simulink model "proc_control_lite"  (R2024b)
settings: Solver=FixedStepAuto  StartTime=0.0  StopTime=inf  RelTol=1e-3
InitFcn:
  | InitProcControl;
StartFcn:
  | LoadParams;
model workspace (MAT data in the model file):
  SL_ROS_VariableLengthArrays_MaxSizes : object (value not decoded)
values from neighbouring files (symbols this model uses):
  A = T200Spec16V{:,3}    [InitProcControl.m]
  N = T200Spec16V{:,6}    [InitProcControl.m]
  PWM = T200Spec16V{:,1}    [InitProcControl.m]
undefined symbols (not defined in the file or in its folder): config, current_gains, DiscIntNeverNeededParam, is_mpc_alive, is_trajectory_done, motor1, motor2, motor3, motor4, motor5, motor6, motor7, motor8, MPC, mpc_mode, mpc_status, orientation, physics, pose, position, simulation, simulink, target_reached, thrusters_status, thrusters_status_SL_Info, twist
libraries: ros2lib x64, dspstat3 x24, aerolibutil x15, dspfdesign x7, simulink x5, mpclib x3, matrix_library x3, robotcorelib x2, sharedtransform x1, sharedTrackingLibrary x1
(part 3 of 3)

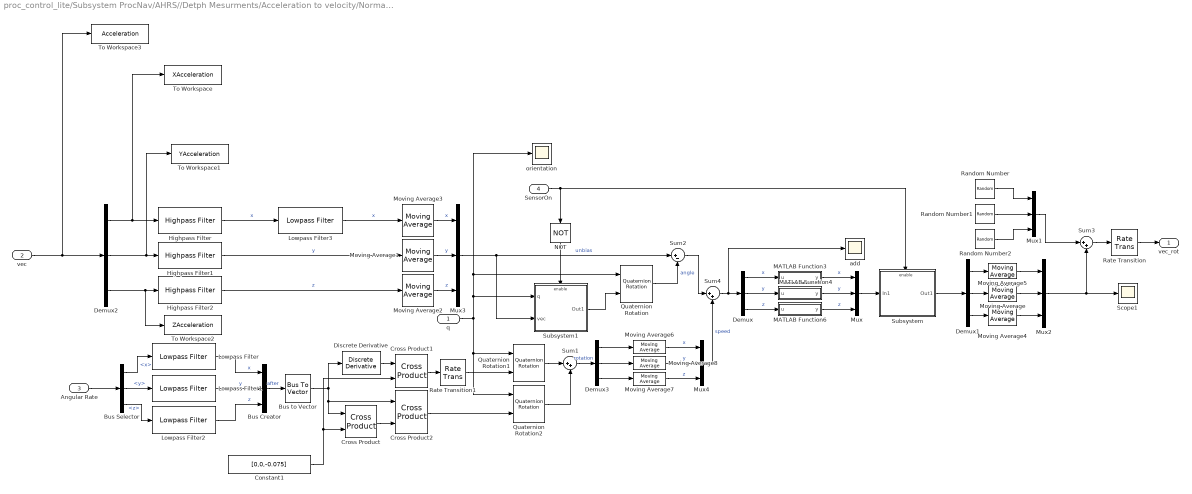
== system proc_control_lite/Subsystem ProcNav/AHRS//Detph Mesurments/Acceleration to velocity/Normal mode ==
  q : Inport
  vec : Inport  Port=2
  Angular Rate : Inport  Port=3
  SensorOn : Inport  Port=4
  Bus Creator : BusCreator  Inputs=3
  Bus Selector : BusSelector  OutputSignals=x,y,z
  Bus to Vector : BusToVector
  Constant1 : Constant  Value=[0,0,-0.075]
  Cross Product : matrix_library/Cross Product
  Cross Product1 : matrix_library/Cross Product
  Cross Product2 : matrix_library/Cross Product
  Demux{,1..3} (4 alike) : Demux  Outputs=3
  Discrete Derivative : simulink/Discrete/Discrete Derivative  gainval=1.0  ICPrevScaledInput=0.0  OutMin=[]  OutMax=[]  OutDataType=fixdt(1, 16)  OutScaling=2^-10  DoSatur=off
  Highpass Filter : dspfdesign/Highpass Filter  FilterType=IIR  DesignForMinimumOrder=on  FilterOrder=50  StopbandFrequency=0.5  PassbandFrequency=0.75  StopbandAttenuation=100  PassbandRipple=0.1  SampleRateMode=Specify on dialog  SampleRate=50  SimulateUsing=Interpreted execution  roundingMode=Floor  coeffsDataTypeStr=fixdt(1,16)
  Highpass Filter1 : dspfdesign/Highpass Filter  FilterType=IIR  DesignForMinimumOrder=on  FilterOrder=50  StopbandFrequency=0.2  PassbandFrequency=0.25  StopbandAttenuation=100  PassbandRipple=0.1  SampleRateMode=Use normalized frequency (0 to 1)  SampleRate=44100  SimulateUsing=Interpreted execution  roundingMode=Floor  coeffsDataTypeStr=fixdt(1,16)
  Highpass Filter2 : dspfdesign/Highpass Filter  FilterType=IIR  DesignForMinimumOrder=on  FilterOrder=50  StopbandFrequency=0.2  PassbandFrequency=0.25  StopbandAttenuation=100  PassbandRipple=0.1  SampleRateMode=Use normalized frequency (0 to 1)  SampleRate=44100  SimulateUsing=Interpreted execution  roundingMode=Floor  coeffsDataTypeStr=fixdt(1,16)
  Lowpass Filter{,1..3} (4 alike) : dspfdesign/Lowpass Filter  FilterType=FIR  DesignForMinimumOrder=on  FilterOrder=50  PassbandFrequency=0.10  StopbandFrequency=0.15  PassbandRipple=0.1  StopbandAttenuation=80  SampleRateMode=Use normalized frequency (0 to 1)  SampleRate=44100  SimulateUsing=Interpreted execution  roundingMode=Floor  coeffsDataTypeStr=fixdt(1,16)
  MATLAB Function3 : MATLAB Function  TreatAsAtomicUnit=on
  MATLAB Function4 : MATLAB Function  TreatAsAtomicUnit=on
  MATLAB Function6 : MATLAB Function  TreatAsAtomicUnit=on
  Moving Average : dspstat3/Moving Average  Method=Sliding window  ForgettingFactorPort=off  SpecifyWindowLength=on  WindowLength=10  OverlapLength=9  AllowArbitraryInputLength=off  ForgettingFactor=0.9  SimulateUsing=Interpreted execution
  Moving Average{1..3,6..8} (6 alike) : dspstat3/Moving Average  Method=Sliding window  ForgettingFactorPort=off  SpecifyWindowLength=on  WindowLength=5  OverlapLength=4  AllowArbitraryInputLength=off  ForgettingFactor=0.9  SimulateUsing=Interpreted execution
  Moving Average4 : dspstat3/Moving Average  Method=Sliding window  ForgettingFactorPort=off  SpecifyWindowLength=on  WindowLength=10  OverlapLength=9  AllowArbitraryInputLength=off  ForgettingFactor=0.9  SimulateUsing=Interpreted execution
  Moving Average5 : dspstat3/Moving Average  Method=Sliding window  ForgettingFactorPort=off  SpecifyWindowLength=on  WindowLength=10  OverlapLength=9  AllowArbitraryInputLength=off  ForgettingFactor=0.9  SimulateUsing=Interpreted execution
  Mux{,1..4} (5 alike) : Mux  Inputs=3
  NOT : Logic  Operator=NOT  IconShape=distinctive  AllPortsSameDT=off  OutDataTypeStr=boolean
  Quaternion Rotation : aerolibutil/Quaternion Rotation
  Quaternion Rotation1 : aerolibutil/Quaternion Rotation
  Quaternion Rotation2 : aerolibutil/Quaternion Rotation
  Random Number : RandomNumber  Variance=0.0000000001  Seed=1  SampleTime=0.02
  Random Number1 : RandomNumber  Variance=0.0000000001  Seed=525886  SampleTime=0.02
  Random Number2 : RandomNumber  Variance=0.0000000001  Seed=4  SampleTime=0.02
  Rate Transition : RateTransition  OutPortSampleTime=0.02
  Rate Transition1 : RateTransition  OutPortSampleTime=0.02
  Scope1 : Scope
  Subsystem : Subsystem
  Subsystem1 : Subsystem
  Sum1 : Sum  Inputs=|++
  Sum2 : Sum  Inputs=|+-
  Sum3 : Sum  Inputs=|++
  Sum4 : Sum  Inputs=|++
  To Workspace : ToWorkspace  VariableName=XAcceleration  SaveFormat=Timeseries  SampleTime=-1
  To Workspace1 : ToWorkspace  VariableName=YAcceleration  SaveFormat=Timeseries  SampleTime=-1
  To Workspace2 : ToWorkspace  VariableName=ZAcceleration  SaveFormat=Timeseries  SampleTime=-1
  To Workspace3 : ToWorkspace  VariableName=Acceleration  SaveFormat=Timeseries  SampleTime=-1
  add : Scope
  orientation : Scope
  vec_rot : Outport
  wires:
  Rate Transition/1 -> vec_rot/1
  Quaternion Rotation1/1 -> Sum1/1
  Cross Product1/1 -> Rate Transition1/1
  Constant1/1 -> Cross Product/2, Cross Product1/2
  Bus to Vector/1 -> Discrete Derivative/1, Cross Product/1, Cross Product2/1
  Discrete Derivative/1 -> Cross Product1/1
  Mux2/1 -> Sum3/2, Scope1/1
  SensorOn/1 -> Subsystem/Enable, NOT/1
  Sum3/1 -> Rate Transition/1
  Subsystem1/1(Out1) -> Quaternion Rotation/2
  NOT/1 -> Subsystem1/Enable
  Mux3/1 -> Subsystem1/2(vec), Sum2/1  "unbias"
  Bus Creator/1 -> Bus to Vector/1  "after"
  Bus Selector/1 -> Lowpass Filter/1  "<x>"
  Bus Selector/2 -> Lowpass Filter1/1  "<y>"
  Bus Selector/3 -> Lowpass Filter2/1  "<z>"
  Mux/1 -> Subsystem/1(In1)
  MATLAB Function6/1(y) -> Mux/3  "z"
  MATLAB Function4/1(y) -> Mux/2  "y"
  MATLAB Function3/1(y) -> Mux/1  "x"
  Random Number/1 -> Mux1/1
  Random Number1/1 -> Mux1/2
  Random Number2/1 -> Mux1/3
  Mux1/1 -> Sum3/1
  Quaternion Rotation/1 -> Sum2/2  "angle"
  Rate Transition1/1 -> Quaternion Rotation1/2
  Cross Product2/1 -> Quaternion Rotation2/2
  Angular Rate/1 -> Bus Selector/1
  Cross Product/1 -> Cross Product2/2
  Quaternion Rotation2/1 -> Sum1/2
  Sum1/1 -> Demux3/1  "rotation"
  Sum2/1 -> Sum4/1
  q/1 -> Quaternion Rotation/1, orientation/1, Subsystem1/1(q), Quaternion Rotation1/1, Quaternion Rotation2/1
  Demux1/1 -> Moving Average5/1
  Subsystem/1(Out1) -> Demux1/1
  Moving Average5/1 -> Mux2/1
  Demux1/2 -> Moving Average/1
  Demux1/3 -> Moving Average4/1
  Moving Average/1 -> Mux2/2
  Moving Average4/1 -> Mux2/3
  vec/1 -> To Workspace3/1, Demux2/1
  Demux2/1 -> To Workspace/1, Highpass Filter/1
  Demux2/2 -> To Workspace1/1, Highpass Filter1/1
  Demux2/3 -> To Workspace2/1, Highpass Filter2/1
  Moving Average2/1 -> Mux3/3  "z"
  Moving Average1/1 -> Mux3/2  "y"
  Moving Average3/1 -> Mux3/1  "x"
  Lowpass Filter1/1 -> Bus Creator/2  "y"
  Lowpass Filter/1 -> Bus Creator/1  "x"
  Lowpass Filter2/1 -> Bus Creator/3  "z"
  Demux/1 -> MATLAB Function3/1(u)  "x"
  Demux/2 -> MATLAB Function4/1(u)  "y"
  Demux/3 -> MATLAB Function6/1(u)  "z"
  Moving Average8/1 -> Mux4/2  "y"
  Demux3/1 -> Moving Average6/1
  Moving Average7/1 -> Mux4/3  "z"
  Demux3/2 -> Moving Average8/1
  Moving Average6/1 -> Mux4/1  "x"
  Demux3/3 -> Moving Average7/1
  Mux4/1 -> Sum4/2  "speed"
  Sum4/1 -> add/1, Demux/1
  Highpass Filter/1 -> Lowpass Filter3/1  "x"
  Highpass Filter1/1 -> Moving Average1/1  "y"
  Highpass Filter2/1 -> Moving Average2/1  "z"
  Lowpass Filter3/1 -> Moving Average3/1  "x"

== system proc_control_lite/Subsystem ProcNav/AHRS//Detph Mesurments/Acceleration to velocity/Simulation ==
  vec : Inport
  Integrator : Integrator
  Rate Transition : RateTransition  OutPortSampleTime=0.02
  vec_rot : Outport
  wires:
  vec/1 -> Integrator/1
  Integrator/1 -> Rate Transition/1
  Rate Transition/1 -> vec_rot/1

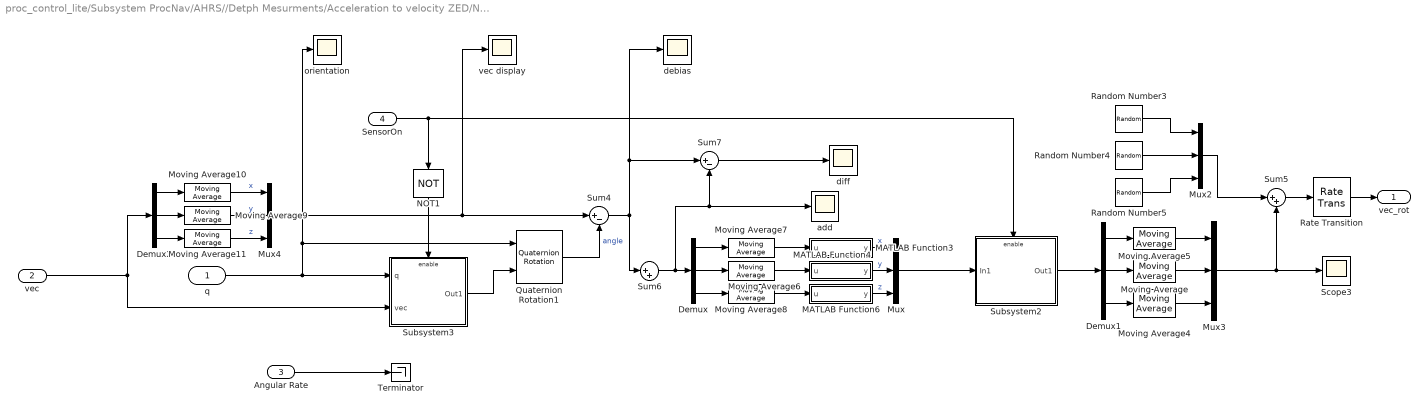
== system proc_control_lite/Subsystem ProcNav/AHRS//Detph Mesurments/Acceleration to velocity ZED/Normal mode ==
  q : Inport
  vec : Inport  Port=2
  Angular Rate : Inport  Port=3
  SensorOn : Inport  Port=4
  Demux : Demux  Outputs=3
  Demux1 : Demux  Outputs=3
  Demux2 : Demux  Outputs=3
  MATLAB Function3 : MATLAB Function  TreatAsAtomicUnit=on
  MATLAB Function4 : MATLAB Function  TreatAsAtomicUnit=on
  MATLAB Function6 : MATLAB Function  TreatAsAtomicUnit=on
  Moving Average : dspstat3/Moving Average  Method=Sliding window  ForgettingFactorPort=off  SpecifyWindowLength=on  WindowLength=10  OverlapLength=9  AllowArbitraryInputLength=off  ForgettingFactor=0.9  SimulateUsing=Interpreted execution
  Moving Average10 : dspstat3/Moving Average  Method=Sliding window  ForgettingFactorPort=off  SpecifyWindowLength=on  WindowLength=25  OverlapLength=24  AllowArbitraryInputLength=off  ForgettingFactor=0.9  SimulateUsing=Interpreted execution
  Moving Average11 : dspstat3/Moving Average  Method=Sliding window  ForgettingFactorPort=off  SpecifyWindowLength=on  WindowLength=25  OverlapLength=24  AllowArbitraryInputLength=off  ForgettingFactor=0.9  SimulateUsing=Interpreted execution
  Moving Average4 : dspstat3/Moving Average  Method=Sliding window  ForgettingFactorPort=off  SpecifyWindowLength=on  WindowLength=10  OverlapLength=9  AllowArbitraryInputLength=off  ForgettingFactor=0.9  SimulateUsing=Interpreted execution
  Moving Average5 : dspstat3/Moving Average  Method=Sliding window  ForgettingFactorPort=off  SpecifyWindowLength=on  WindowLength=10  OverlapLength=9  AllowArbitraryInputLength=off  ForgettingFactor=0.9  SimulateUsing=Interpreted execution
  Moving Average6 : dspstat3/Moving Average  Method=Sliding window  ForgettingFactorPort=off  SpecifyWindowLength=on  WindowLength=5  OverlapLength=4  AllowArbitraryInputLength=off  ForgettingFactor=0.9  SimulateUsing=Interpreted execution
  Moving Average7 : dspstat3/Moving Average  Method=Sliding window  ForgettingFactorPort=off  SpecifyWindowLength=on  WindowLength=5  OverlapLength=4  AllowArbitraryInputLength=off  ForgettingFactor=0.9  SimulateUsing=Interpreted execution
  Moving Average8 : dspstat3/Moving Average  Method=Sliding window  ForgettingFactorPort=off  SpecifyWindowLength=on  WindowLength=5  OverlapLength=4  AllowArbitraryInputLength=off  ForgettingFactor=0.9  SimulateUsing=Interpreted execution
  Moving Average9 : dspstat3/Moving Average  Method=Sliding window  ForgettingFactorPort=off  SpecifyWindowLength=on  WindowLength=25  OverlapLength=24  AllowArbitraryInputLength=off  ForgettingFactor=0.9  SimulateUsing=Interpreted execution
  Mux{,2..4} (4 alike) : Mux  Inputs=3
  NOT1 : Logic  Operator=NOT  IconShape=distinctive  AllPortsSameDT=off  OutDataTypeStr=boolean
  Quaternion Rotation1 : aerolibutil/Quaternion Rotation
  Random Number3 : RandomNumber  Variance=0.000000000000000000001  Seed=1  SampleTime=0.02
  Random Number4 : RandomNumber  Variance=0.000000000000000000001  Seed=525886  SampleTime=0.02
  Random Number5 : RandomNumber  Variance=0.000000000000000000001  Seed=645156145645445  SampleTime=0.02
  Rate Transition : RateTransition  OutPortSampleTime=0.02
  Scope3 : Scope
  Subsystem2 : Subsystem
  Subsystem3 : Subsystem
  Sum4 : Sum  Inputs=|+-
  Sum5 : Sum  Inputs=|++
  Sum6 : Sum  Inputs=|++
  Sum7 : Sum  Inputs=|+-
  Terminator : Terminator
  add : Scope
  debias : Scope
  diff : Scope
  orientation : Scope
  vec display : Scope
  vec_rot : Outport
  wires:
  Moving Average7/1 -> MATLAB Function3/1(u)
  vec/1 -> Demux2/1, Subsystem3/2(vec)
  Moving Average6/1 -> MATLAB Function4/1(u)
  Demux2/3 -> Moving Average11/1
  Sum4/1 -> Sum6/1, Sum7/1, debias/1
  Sum7/1 -> diff/1
  Demux/1 -> Moving Average7/1
  Moving Average/1 -> Mux3/2
  Subsystem3/1(Out1) -> Quaternion Rotation1/2
  Sum5/1 -> Rate Transition/1
  Moving Average10/1 -> Mux4/1  "x"
  Subsystem2/1(Out1) -> Demux1/1
  SensorOn/1 -> Subsystem2/Enable, NOT1/1
  Demux/2 -> Moving Average6/1
  Mux3/1 -> Sum5/2, Scope3/1
  Moving Average4/1 -> Mux3/3
  q/1 -> orientation/1, Quaternion Rotation1/1, Subsystem3/1(q)
  Demux1/2 -> Moving Average/1
  NOT1/1 -> Subsystem3/Enable
  Demux2/2 -> Moving Average9/1
  Moving Average5/1 -> Mux3/1
  Demux1/1 -> Moving Average5/1
  Moving Average11/1 -> Mux4/3  "z"
  Mux4/1 -> vec display/1, Sum4/1
  MATLAB Function6/1(y) -> Mux/3  "z"
  Demux2/1 -> Moving Average10/1
  Random Number3/1 -> Mux2/1
  Random Number4/1 -> Mux2/2
  Moving Average8/1 -> MATLAB Function6/1(u)
  Moving Average9/1 -> Mux4/2  "y"
  Random Number5/1 -> Mux2/3
  Demux1/3 -> Moving Average4/1
  Sum6/1 -> add/1, Sum7/2, Demux/1
  Rate Transition/1 -> vec_rot/1
  MATLAB Function4/1(y) -> Mux/2  "y"
  MATLAB Function3/1(y) -> Mux/1  "x"
  Quaternion Rotation1/1 -> Sum4/2  "angle"
  Mux2/1 -> Sum5/1
  Demux/3 -> Moving Average8/1
  Mux/1 -> Subsystem2/1(In1)
  Angular Rate/1 -> Terminator/1

== system proc_control_lite/Subsystem ProcNav/AHRS//Detph Mesurments/Acceleration to velocity ZED/Subsystem1 ==
  vec : Inport
  Integrator : Integrator
  Rate Transition : RateTransition  OutPortSampleTime=0.02
  vec_rot : Outport
  wires:
  vec/1 -> Integrator/1
  Integrator/1 -> Rate Transition/1
  Rate Transition/1 -> vec_rot/1

== system proc_control_lite/Subsystem ProcNav/DVL Measurements/DVL2Ship/Enabled Subsystem ==
  dvl Rotation : Inport
  Enable : EnablePort
  Rotation Angles to Quaternions : sharedtransform/Rotation Angles to Quaternions  rotationOrder=XYZ  aMode=aMode
  Quat : Outport
  wires:
  dvl Rotation/1 -> Rotation Angles to Quaternions/1
  Rotation Angles to Quaternions/1 -> Quat/1

== system proc_control_lite/Subsystem Trajectory/singleWpts Trajectory Control DEBUG only/Resettable Subsystem/Subsystem ==
  In1 : Inport
  linWpts : Inport  Port=2
  time : Inport  Port=3
  Polynomial Trajectory : robotcorelib/Polynomial Trajectory  WaypointSource=External  Waypoints=[ 0, 2, 1, 5, 0; -1, 3, 1, 4, 4 ]  TimePoints=[ 0, 1, 2, 3, 4 ]  TimeInterval=[ 1, 4 ]  Method=Cubic Polynomial  ParameterSource=Internal  VelocityBoundaryCondition=zeros( 3, 2 )  AccelerationBoundaryCondition=zeros( 2, 5 )  SimulateUsing=Code generation
  Terminator : Terminator
  n1 : Outport
  v1 : Outport  Port=2
  wires:
  In1/1 -> Polynomial Trajectory/1
  linWpts/1 -> Polynomial Trajectory/2
  time/1 -> Polynomial Trajectory/3
  Polynomial Trajectory/1 -> n1/1
  Polynomial Trajectory/2 -> v1/1
  Polynomial Trajectory/3 -> Terminator/1

== system proc_control_lite/Ros Command/Get_ROS_param/MPC Parameters/MPC Gains/Gains Default ==
  Bus Creator : BusCreator  Inputs=3
  MATLAB System1 : MATLABSystem  System=Vector2DoubleArray  arraySize=[1 MPC.nu]  constantName='Default MVR'  SimulateUsing=Code generation
      mask Type: Vector2DoubleArray
      mask Display:
      | disp('Vector2DoubleArray');
      | port_label('input',1,'vector');
      | port_label('input',2,'length');
      | port_label('output',1,'array');
  MATLAB System3 : MATLABSystem  System=Vector2DoubleArray  arraySize=[1 MPC.nx]  constantName='Default OV'  SimulateUsing=Code generation
      mask Type: Vector2DoubleArray
      mask Display:
      | disp('Vector2DoubleArray');
      | port_label('input',1,'vector');
      | port_label('input',2,'length');
      | port_label('output',1,'array');
  MATLAB System4 : MATLABSystem  System=Vector2DoubleArray  arraySize=[1, MPC.nu]  constantName='Default MV'  SimulateUsing=Code generation
      mask Type: Vector2DoubleArray
      mask Display:
      | disp('Vector2DoubleArray');
      | port_label('input',1,'vector');
      | port_label('input',2,'length');
      | port_label('output',1,'array');
  MV : ros2lib/Get Parameter  ParameterName=proc_control.mpc.gains.default.mv  ParameterType=double[]  ParameterMaxArrayLength=64  ParameterInitialValue=double([30,30,30,45,45,45,45,0])  SampleTime=-1  ModelName=proc_control_lite  BlockId=ParamGet_proc_control_lite_72
  MVR : ros2lib/Get Parameter  ParameterName=proc_control.mpc.gains.default.mvr  ParameterType=double[]  ParameterMaxArrayLength=64  ParameterInitialValue=double([30,30,30,45,45,45,45,0])  SampleTime=-1  ModelName=proc_control_lite  BlockId=ParamGet_proc_control_lite_74
  OV : ros2lib/Get Parameter  ParameterName=proc_control.mpc.gains.default.ov  ParameterType=double[]  ParameterMaxArrayLength=64  ParameterInitialValue=double([30.0,30.0,30.0,45.0,45.0,45.0,45.0,0.0,0.0,0.0,0.0,0.0,0.0])  SampleTime=-1  ModelName=proc_control_lite  BlockId=ParamGet_proc_control_lite_66
  default : Outport
  wires:
  OV/1 -> MATLAB System3/1
  OV/2 -> MATLAB System3/2
  MVR/2 -> MATLAB System1/2
  MV/1 -> MATLAB System4/1
  MATLAB System3/1 -> Bus Creator/1  "OV"
  MV/2 -> MATLAB System4/2
  MATLAB System4/1 -> Bus Creator/2  "MV"
  MVR/1 -> MATLAB System1/1
  MATLAB System1/1 -> Bus Creator/3  "MVR"
  Bus Creator/1 -> default/1  "predefined"

== system proc_control_lite/Ros Command/Get_ROS_param/MPC Parameters/MPC Gains/Gains Mode 10 ==
  Bus Creator : BusCreator  Inputs=3
  MATLAB System3 : MATLABSystem  System=Vector2DoubleArray  arraySize=[1 MPC.nu]  constantName='M10 MVR'  SimulateUsing=Code generation
      mask Type: Vector2DoubleArray
      mask Display:
      | disp('Vector2DoubleArray');
      | port_label('input',1,'vector');
      | port_label('input',2,'length');
      | port_label('output',1,'array');
  MATLAB System4 : MATLABSystem  System=Vector2DoubleArray  arraySize=[1 MPC.nx]  constantName='M10 OV'  SimulateUsing=Code generation
      mask Type: Vector2DoubleArray
      mask Display:
      | disp('Vector2DoubleArray');
      | port_label('input',1,'vector');
      | port_label('input',2,'length');
      | port_label('output',1,'array');
  MATLAB System5 : MATLABSystem  System=Vector2DoubleArray  arraySize=[1 MPC.nu]  constantName='M10 MV'  SimulateUsing=Code generation
      mask Type: Vector2DoubleArray
      mask Display:
      | disp('Vector2DoubleArray');
      | port_label('input',1,'vector');
      | port_label('input',2,'length');
      | port_label('output',1,'array');
  MV : ros2lib/Get Parameter  ParameterName=proc_control.mpc.gains.c10.mv  ParameterType=double[]  ParameterMaxArrayLength=64  ParameterInitialValue=uint8([30,30,30,45,45,45,45,0])  SampleTime=-1  ModelName=proc_control_lite  BlockId=ParamGet_proc_control_lite_98
  MVR : ros2lib/Get Parameter  ParameterName=proc_control.mpc.gains.c10.mvr  ParameterType=double[]  ParameterMaxArrayLength=64  ParameterInitialValue=uint8([30,30,30,45,45,45,45,0])  SampleTime=-1  ModelName=proc_control_lite  BlockId=ParamGet_proc_control_lite_99
  OV : ros2lib/Get Parameter  ParameterName=proc_control.mpc.gains.c10.ov  ParameterType=double[]  ParameterMaxArrayLength=64  ParameterInitialValue=uint8([30,30,30,45,45,45,45,0,0,0,0,0,0])  SampleTime=-1  ModelName=proc_control_lite  BlockId=ParamGet_proc_control_lite_97
  c10 : Outport
  wires:
  OV/1 -> MATLAB System4/1
  OV/2 -> MATLAB System4/2
  MVR/2 -> MATLAB System3/2
  MV/1 -> MATLAB System5/1
  MATLAB System4/1 -> Bus Creator/1  "OV"
  MV/2 -> MATLAB System5/2
  MATLAB System5/1 -> Bus Creator/2  "MV"
  MVR/1 -> MATLAB System3/1
  MATLAB System3/1 -> Bus Creator/3  "MVR"
  Bus Creator/1 -> c10/1  "c10"

== system proc_control_lite/Ros Command/Get_ROS_param/MPC Parameters/MPC Gains/Gains Mode 11 ==
  Bus Creator : BusCreator  Inputs=3
  MATLAB System3 : MATLABSystem  System=Vector2DoubleArray  arraySize=[1 MPC.nu]  constantName='M11 MVR'  SimulateUsing=Code generation
      mask Type: Vector2DoubleArray
      mask Display:
      | disp('Vector2DoubleArray');
      | port_label('input',1,'vector');
      | port_label('input',2,'length');
      | port_label('output',1,'array');
  MATLAB System4 : MATLABSystem  System=Vector2DoubleArray  arraySize=[1 MPC.nx]  constantName='M11 OV'  SimulateUsing=Code generation
      mask Type: Vector2DoubleArray
      mask Display:
      | disp('Vector2DoubleArray');
      | port_label('input',1,'vector');
      | port_label('input',2,'length');
      | port_label('output',1,'array');
  MATLAB System5 : MATLABSystem  System=Vector2DoubleArray  arraySize=[1 MPC.nu]  constantName='M11 MV'  SimulateUsing=Code generation
      mask Type: Vector2DoubleArray
      mask Display:
      | disp('Vector2DoubleArray');
      | port_label('input',1,'vector');
      | port_label('input',2,'length');
      | port_label('output',1,'array');
  MV : ros2lib/Get Parameter  ParameterName=proc_control.mpc.gains.c11.mv  ParameterType=double[]  ParameterMaxArrayLength=64  ParameterInitialValue=uint8([30,30,30,45,45,45,45,0])  SampleTime=-1  ModelName=proc_control_lite  BlockId=ParamGet_proc_control_lite_107
  MVR : ros2lib/Get Parameter  ParameterName=proc_control.mpc.gains.c11.mvr  ParameterType=double[]  ParameterMaxArrayLength=64  ParameterInitialValue=uint8([30,30,30,45,45,45,45,0])  SampleTime=-1  ModelName=proc_control_lite  BlockId=ParamGet_proc_control_lite_108
  OV : ros2lib/Get Parameter  ParameterName=proc_control.mpc.gains.c11.ov  ParameterType=double[]  ParameterMaxArrayLength=64  ParameterInitialValue=uint8([30,30,30,45,45,45,45,0,0,0,0,0,0])  SampleTime=-1  ModelName=proc_control_lite  BlockId=ParamGet_proc_control_lite_106
  c11 : Outport
  wires:
  OV/1 -> MATLAB System4/1
  OV/2 -> MATLAB System4/2
  MVR/2 -> MATLAB System3/2
  MV/1 -> MATLAB System5/1
  MATLAB System4/1 -> Bus Creator/1  "OV"
  MV/2 -> MATLAB System5/2
  MATLAB System5/1 -> Bus Creator/2  "MV"
  MVR/1 -> MATLAB System3/1
  MATLAB System3/1 -> Bus Creator/3  "MVR"
  Bus Creator/1 -> c11/1  "c11"

== system proc_control_lite/Ros Command/Get_ROS_param/MPC Parameters/MPC Gains/Gains Mode 19 ==
  Bus Creator : BusCreator  Inputs=3
  MATLAB System3 : MATLABSystem  System=Vector2DoubleArray  arraySize=[1 MPC.nu]  constantName='M19 MVR'  SimulateUsing=Code generation
      mask Type: Vector2DoubleArray
      mask Display:
      | disp('Vector2DoubleArray');
      | port_label('input',1,'vector');
      | port_label('input',2,'length');
      | port_label('output',1,'array');
  MATLAB System4 : MATLABSystem  System=Vector2DoubleArray  arraySize=[1 MPC.nx]  constantName='M19 OV'  SimulateUsing=Code generation
      mask Type: Vector2DoubleArray
      mask Display:
      | disp('Vector2DoubleArray');
      | port_label('input',1,'vector');
      | port_label('input',2,'length');
      | port_label('output',1,'array');
  MATLAB System5 : MATLABSystem  System=Vector2DoubleArray  arraySize=[1 MPC.nu]  constantName='M19 MV'  SimulateUsing=Code generation
      mask Type: Vector2DoubleArray
      mask Display:
      | disp('Vector2DoubleArray');
      | port_label('input',1,'vector');
      | port_label('input',2,'length');
      | port_label('output',1,'array');
  MV : ros2lib/Get Parameter  ParameterName=proc_control.mpc.gains.c19.mv  ParameterType=double[]  ParameterMaxArrayLength=64  ParameterInitialValue=uint8([30,30,30,45,45,45,45,0])  SampleTime=-1  ModelName=proc_control_lite  BlockId=ParamGet_proc_control_lite_116
  MVR : ros2lib/Get Parameter  ParameterName=proc_control.mpc.gains.c19.mvr  ParameterType=double[]  ParameterMaxArrayLength=64  ParameterInitialValue=uint8([30,30,30,45,45,45,45,0])  SampleTime=-1  ModelName=proc_control_lite  BlockId=ParamGet_proc_control_lite_117
  OV : ros2lib/Get Parameter  ParameterName=proc_control.mpc.gains.c19.ov  ParameterType=double[]  ParameterMaxArrayLength=64  ParameterInitialValue=uint8([30,30,30,45,45,45,45,0,0,0,0,0,0])  SampleTime=-1  ModelName=proc_control_lite  BlockId=ParamGet_proc_control_lite_115
  c19 : Outport
  wires:
  OV/1 -> MATLAB System4/1
  OV/2 -> MATLAB System4/2
  MVR/2 -> MATLAB System3/2
  MV/1 -> MATLAB System5/1
  MATLAB System4/1 -> Bus Creator/1  "OV"
  MV/2 -> MATLAB System5/2
  MATLAB System5/1 -> Bus Creator/2  "MV"
  MVR/1 -> MATLAB System3/1
  MATLAB System3/1 -> Bus Creator/3  "MVR"
  Bus Creator/1 -> c19/1  "c19"

== system proc_control_lite/Ros Command/Get_ROS_param/MPC Parameters/MPC Gains/Gains No DVL ==
  Bus Creator : BusCreator  Inputs=1
  MATLAB System5 : MATLABSystem  System=Vector2DoubleArray  arraySize=[1 MPC.nu]  constantName='No DVL MV'  SimulateUsing=Code generation
      mask Type: Vector2DoubleArray
      mask Display:
      | disp('Vector2DoubleArray');
      | port_label('input',1,'vector');
      | port_label('input',2,'length');
      | port_label('output',1,'array');
  MV : ros2lib/Get Parameter  ParameterName=proc_control.mpc.gains.noDvl.mv  ParameterType=double[]  ParameterMaxArrayLength=64  ParameterInitialValue=uint8([30,30,30,45,45,45,45,0])  SampleTime=-1  ModelName=proc_control_lite  BlockId=ParamGet_proc_control_lite_133
  noDvl : Outport
  wires:
  MV/2 -> MATLAB System5/2
  MV/1 -> MATLAB System5/1
  MATLAB System5/1 -> Bus Creator/1  "MV"
  Bus Creator/1 -> noDvl/1  "noDvl"

== system proc_control_lite/Subsystem ProcNav/AHRS//Detph Mesurments/Acceleration to velocity/Normal mode/Subsystem ==
  In1 : Inport
  SensorOn : EnablePort
  Discrete-Time Integrator : DiscreteIntegrator  IntegratorMethod=Integration: Trapezoidal  InitialCondition=[0,0,0]  SampleTime=0.02  ICPrevOutput=DiscIntNeverNeededParam  ICPrevScaledInput=DiscIntNeverNeededParam
  Out1 : Outport
  wires:
  Discrete-Time Integrator/1 -> Out1/1
  In1/1 -> Discrete-Time Integrator/1

== system proc_control_lite/Subsystem ProcNav/AHRS//Detph Mesurments/Acceleration to velocity/Normal mode/Subsystem1 ==
  q : Inport
  vec : Inport  Port=2
  SensorOn : EnablePort
  Demux : Demux  Outputs=3
  Moving Average : dspstat3/Moving Average  Method=Sliding window  ForgettingFactorPort=off  SpecifyWindowLength=on  WindowLength=50  OverlapLength=49  AllowArbitraryInputLength=off  ForgettingFactor=0.9  SimulateUsing=Interpreted execution
  Moving Average1 : dspstat3/Moving Average  Method=Sliding window  ForgettingFactorPort=off  SpecifyWindowLength=on  WindowLength=50  OverlapLength=49  AllowArbitraryInputLength=off  ForgettingFactor=0.9  SimulateUsing=Interpreted execution
  Moving Average2 : dspstat3/Moving Average  Method=Sliding window  ForgettingFactorPort=off  SpecifyWindowLength=on  WindowLength=50  OverlapLength=49  AllowArbitraryInputLength=off  ForgettingFactor=0.9  SimulateUsing=Interpreted execution
  Mux : Mux  Inputs=3
  Quaternion Inverse : aerolibutil/Quaternion Inverse
  Quaternion Rotation : aerolibutil/Quaternion Rotation
  Out1 : Outport
  wires:
  vec/1 -> Quaternion Rotation/2
  Moving Average/1 -> Mux/2
  Moving Average2/1 -> Mux/1
  Moving Average1/1 -> Mux/3
  Mux/1 -> Out1/1
  Quaternion Rotation/1 -> Demux/1
  q/1 -> Quaternion Inverse/1
  Quaternion Inverse/1 -> Quaternion Rotation/1  "qS2W"
  Demux/3 -> Moving Average1/1
  Demux/1 -> Moving Average2/1
  Demux/2 -> Moving Average/1

== system proc_control_lite/Subsystem ProcNav/AHRS//Detph Mesurments/Acceleration to velocity ZED/Normal mode/Subsystem2 ==
  In1 : Inport
  SensorOn : EnablePort
  Discrete-Time Integrator : DiscreteIntegrator  IntegratorMethod=Integration: Trapezoidal  InitialCondition=[0,0,0]  SampleTime=0.02  ICPrevOutput=DiscIntNeverNeededParam  ICPrevScaledInput=DiscIntNeverNeededParam
  Out1 : Outport
  wires:
  Discrete-Time Integrator/1 -> Out1/1
  In1/1 -> Discrete-Time Integrator/1

== system proc_control_lite/Subsystem ProcNav/AHRS//Detph Mesurments/Acceleration to velocity ZED/Normal mode/Subsystem3 ==
  q : Inport
  vec : Inport  Port=2
  SensorOn : EnablePort
  Demux : Demux  Outputs=3
  Moving Average : dspstat3/Moving Average  Method=Sliding window  ForgettingFactorPort=off  SpecifyWindowLength=on  WindowLength=50  OverlapLength=49  AllowArbitraryInputLength=off  ForgettingFactor=0.9  SimulateUsing=Interpreted execution
  Moving Average1 : dspstat3/Moving Average  Method=Sliding window  ForgettingFactorPort=off  SpecifyWindowLength=on  WindowLength=50  OverlapLength=49  AllowArbitraryInputLength=off  ForgettingFactor=0.9  SimulateUsing=Interpreted execution
  Moving Average2 : dspstat3/Moving Average  Method=Sliding window  ForgettingFactorPort=off  SpecifyWindowLength=on  WindowLength=50  OverlapLength=49  AllowArbitraryInputLength=off  ForgettingFactor=0.9  SimulateUsing=Interpreted execution
  Mux : Mux  Inputs=3
  Quaternion Inverse : aerolibutil/Quaternion Inverse
  Quaternion Rotation : aerolibutil/Quaternion Rotation
  Out1 : Outport
  wires:
  vec/1 -> Quaternion Rotation/2
  Moving Average/1 -> Mux/2
  Moving Average2/1 -> Mux/1
  Moving Average1/1 -> Mux/3
  Mux/1 -> Out1/1
  Quaternion Rotation/1 -> Demux/1
  q/1 -> Quaternion Inverse/1
  Quaternion Inverse/1 -> Quaternion Rotation/1  "qS2W"
  Demux/3 -> Moving Average1/1
  Demux/1 -> Moving Average2/1
  Demux/2 -> Moving Average/1

== matlab function proc_control_lite/Subsystem ProcNav/AHRS//Detph Mesurments/Acceleration to velocity/Normal mode/MATLAB Function3 ==
  data: u input; y output
function y = fcn(u)

if (-0.2<u && u<0.2)
    y = 0;
else
    y = u;
end

== matlab function proc_control_lite/Subsystem ProcNav/AHRS//Detph Mesurments/Acceleration to velocity/Normal mode/MATLAB Function4 ==
  data: u input; y output
function y = fcn(u)

if (-0.05<u && u<0.05)
    y = 0;
else
    y = u;
end

== matlab function proc_control_lite/Subsystem ProcNav/AHRS//Detph Mesurments/Acceleration to velocity/Normal mode/MATLAB Function6 ==
  data: u input; y output
function y = fcn(u)

if (-0.05<u && u<0.05)
    y = 0;
else
    y = u;
end

== matlab function proc_control_lite/Subsystem ProcNav/AHRS//Detph Mesurments/MATLAB Function ==
  data: u input; y output
function y = Normalize(u)

%Normailse le quaternions pour éviter la distortions crée par l'erreur de
% de l'intégration.
%q=quaternion(u(1), u(2), u(3), u(4));
d=norm(u);
n=u/d;
if isnan(n)
    y=[1;0;0;0];
else
    y = n;
end

== matlab function proc_control_lite/Subsystem ProcNav/AHRS//Detph Mesurments/Acceleration to velocity ZED/Normal mode/MATLAB Function3 ==
  data: u input; y output
function y = fcn(u)

if (-0.5<u && u<0.5)
    y = 0;
else
    y = u;
end

== matlab function proc_control_lite/Subsystem ProcNav/DVL Measurements/MATLAB Function ==
  data: vBot input; v output; vWater input; thres input; error output; enable output
function [v, error, enable] = DVLManager(vBot,vWater,thres)

    if max(abs(vBot(1:3)))< thres
        %retouner les vitesse du bottom tracking (normal)
        v = vBot(1:3);
        enable = 1;
        error = ones(1,3) * vBot(4);
    elseif max(abs(vWater))< thres
        % retouner les vitesse du water profiling si bottom tracking fail
        v = vWater(1:3);
        enable = 0;
        error = ones(1,3) * vWater(4);
    else
        % Désactiver le dvl si mauvais data
        v = zeros(3,1);
        v(3)= 0;% patch(2);
        enable = 0;
        error = ones(1,3) * vBot(4);
    end
end

== matlab function proc_control_lite/Subsystem Trajectory/SpaceNav/MATLAB Function ==
  data: matrix input; y output; p input
function y = fcn(matrix,p)
%matrix(10)=-matrix(10);
y = repmat(matrix,10,1);

== matlab function proc_control_lite/Subsystem Trajectory/IDLE/MATLAB Function ==
  data: matrix input; y output; p input
function y = fcn(matrix,p)
matrix(10)=-matrix(10);
y = repmat(matrix,10,1);

== matlab function proc_control_lite/Subsystem Controller/Controller List/If Action Subsystem1/MATLAB Function ==
  data: u input; A output; ysec input; Ts input; M input; x input; B output; C output; D output; U output; Y output; X output; DX output
function [A,B,C,D,U,Y,X,DX] = LtvTrimPlantQuat(u,ysec,Ts,M,x)

% Déterminer les dimentions
    nx = size(ysec,2);
    nu = size(u,2);
    p = size(u,1);

% Initialiser les matrices
    A = zeros(nx, nx, p);
    B = zeros(nx, nu, p);
    C = zeros(nx, nx, p);
    D = zeros(nx, nu, p);
    U = zeros(nu, 1, p);
    Y = zeros(13, 1, p);
    X = zeros(13, 1, p);
    DX = zeros(13, 1, p);
    
    
    xkk = x;
for i=1:p
    
    % Actualiser les états
        %xk=ysec(i,:).';
       
            xk=xkk;
      
        
        uk=u(i,:).';
        
    % Lineariser le model dynamique
        [Ac, Bc, C(:,:,i), D(:,:,i)]=AUV8QuatJacobianMatrix(xk,uk);


    % Generate discrete-time model
        A(:,:,i) = expm(Ac*Ts); % Fossen(2021) Eq B.10/B.9 page 662

        BT = Ac(8:13,8:13)\(A(8:13,8:13)-eye(6))*Bc(8:13,1:8); % Fossen(2021) Eq B.11 p 662
        B(:,:,i) = [zeros(7,8); BT];

    % Compute F(x(k+1),u)
       % xkk = ysec()
        % Intégration avec Euler Explicite
        for j=1:M 
          xkk = xkk + AUV8QuatSimFcn(xkk,uk)*(Ts/M);  
          % correct Quaternion
          d=norm(xkk(4:7));
          xkk(4:7) = xkk(4:7)./d;
        end

    % Nominal conditions for discrete-time plant
        U(:,:,i)  = uk.';
        Y(:,:,i)  = xk.';%(Cc*x + Dc*u).';
        X(:,:,i)  = xk.';
        DX(:,:,i) = (xkk-xk).' ;
       
end
disp(X)
end

== matlab function proc_control_lite/Ros Command/Get_ROS_param/Physics Constants/MATLAB Function ==
  data: vec input; array output; length input
function array= fcn(vec, length)
array = zeros(8,6);
for i=1 : 8
    base_index = ((i-1)*6);
    array(i,:) = vec(base_index+1:base_index+6);
end

== matlab function proc_control_lite/Subsystem ProcNav/AHRS//Detph Mesurments/MATLAB Function1 ==
  data: u input; y output
function y = Normalize(u)

%Normailse le quaternions pour éviter la distortions crée par l'erreur de
% de l'intégration.
%q=quaternion(u(1), u(2), u(3), u(4));
d=norm(u);
n=u/d;
if isnan(n)
    y=[1;0;0;0];
else
    y = n;
end

== matlab function proc_control_lite/Subsystem ProcNav/AHRS//Detph Mesurments/Acceleration to velocity ZED/Normal mode/MATLAB Function4 ==
  data: u input; y output
function y = fcn(u)

if (-0.5<u && u<0.5)
    y = 0;
else
    y = u;
end

== matlab function proc_control_lite/Subsystem ProcNav/AHRS//Detph Mesurments/Acceleration to velocity ZED/Normal mode/MATLAB Function6 ==
  data: u input; y output
function y = fcn(u)

if (-0.5<u && u<0.5)
    y = 0;
else
    y = u;
end
